simulink model "INP_test"  (R2024b)
settings: Solver=VariableStepAuto  StartTime=0.0  StopTime=10.0  RelTol=1e-3
libraries: simulink x1, INP x1
settings Model: Creator=blatak  LastModifiedBy=blatak

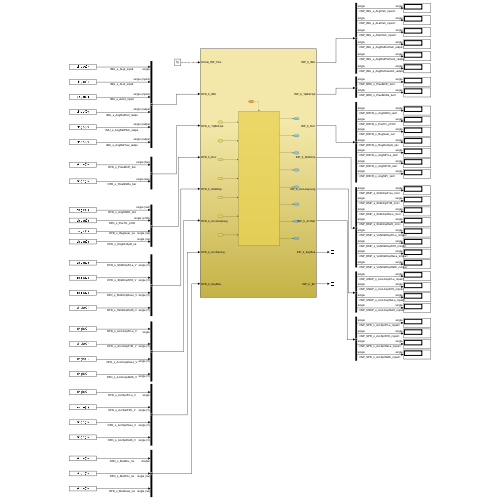
[thumbnail: Simulink's stored preview of the top-level diagram]
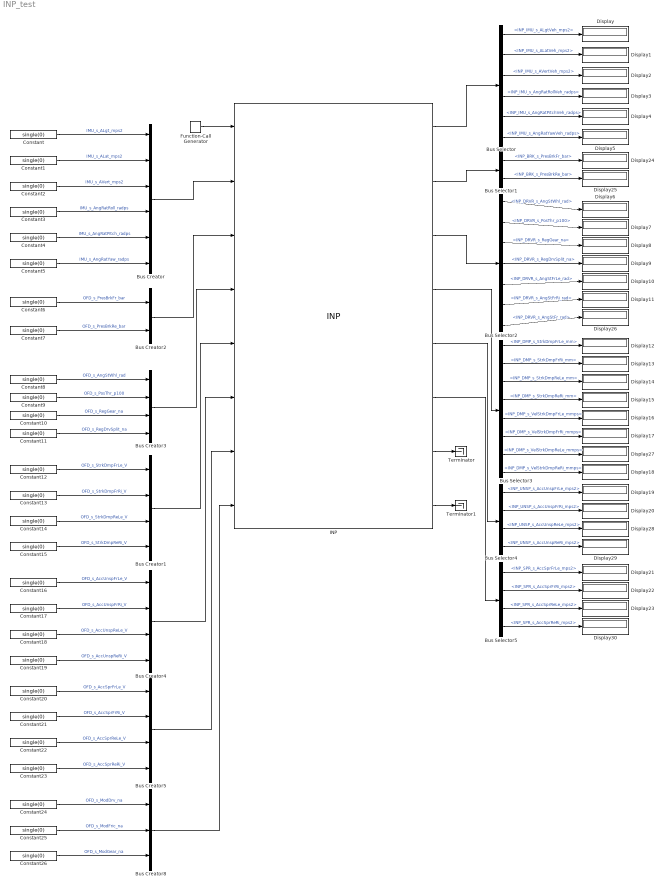
== system INP_test ==
  Bus Creator : BusCreator  Inputs=6  OutDataTypeStr=Bus: OFD_b_IMU
      settings: InheritFromInputs=off
  Bus Creator1 : BusCreator  Inputs=4  OutDataTypeStr=Bus: OFD_b_StrkDmp
      settings: InheritFromInputs=off
  Bus Creator2 : BusCreator  Inputs=2  OutDataTypeStr=Bus: OFD_b_TqBrkHyd
      settings: InheritFromInputs=off
  Bus Creator3 : BusCreator  Inputs=4  OutDataTypeStr=Bus: OFD_b_Drvr
      settings: InheritFromInputs=off
  Bus Creator4 : BusCreator  Inputs=4  OutDataTypeStr=Bus: OFD_b_AccUnsp
      settings: InheritFromInputs=off
  Bus Creator5 : BusCreator  Inputs=4  OutDataTypeStr=Bus: OFD_b_AccSpr
      settings: InheritFromInputs=off
  Bus Creator8 : BusCreator  Inputs=3  OutDataTypeStr=Bus: OFD_b_KeyBoa
      settings: InheritFromInputs=off
  Bus Selector : BusSelector  OutputSignals=INP_IMU_s_ALgtVeh_mps2,INP_IMU_s_ALatVeh_mps2,INP_IMU_s_AVertVeh_mps2,INP_IMU_s_AngRatRollVeh_radps,INP_IMU_s_AngRatPitchVeh_radps,INP_IMU_s_AngRatYawVeh_radps
  Bus Selector1 : BusSelector  OutputSignals=INP_BRK_s_PresBrkFr_bar,INP_BRK_s_PresBrkRe_bar
  Bus Selector2 : BusSelector  OutputSignals=INP_DRVR_s_AngStWhl_rad,INP_DRVR_s_PosThr_p100,INP_DRVR_s_RegGear_na,INP_DRVR_s_RegDrvSplit_na,INP_DRVR_s_AngStFrLe_rad,INP_DRVR_s_AngStFrRi_rad,INP_DRVR_s_AngStFr_rad
  Bus Selector3 : BusSelector  OutputSignals=INP_DMP_s_StrkDmpFrLe_mm,INP_DMP_s_StrkDmpFrRi_mm,INP_DMP_s_StrkDmpReLe_mm,INP_DMP_s_StrkDmpReRi_mm,INP_DMP_s_VelStrkDmpFrLe_mmps,INP_DMP_s_VelStrkDmpFrRi_mmps,INP_DMP_s_VelStrkDmpReLe_mmps,INP_DMP_s_VelStrkDmpReRi_mmps
  Bus Selector4 : BusSelector  OutputSignals=INP_UNSP_s_AccUnspFrLe_mps2,INP_UNSP_s_AccUnspFrRi_mps2,INP_UNSP_s_AccUnspReLe_mps2,INP_UNSP_s_AccUnspReRi_mps2
  Bus Selector5 : BusSelector  OutputSignals=INP_SPR_s_AccSprFrLe_mps2,INP_SPR_s_AccSprFrRi_mps2,INP_SPR_s_AccSprReLe_mps2,INP_SPR_s_AccSprReRi_mps2
  Constant{,1..26} (27 alike) : Constant  Value=single(0)
  Display{,1..30} (31 alike) : Display
  Function-Call Generator : simulink/Ports & Subsystems/Function-Call Generator  sample_time=0.005  numberOfIterations=1  DisallowWideOutput=off
  INP : INP/INP  SystemSampleTime=-1  VariantActivationTime=update diagram  AllowFlexibleInterface=on  Latency=0  AutoFrameSizeCalculation=off
  Terminator : Terminator
  Terminator1 : Terminator
  wires:
  Function-Call Generator/1 -> INP/1
  Constant19/1 -> Bus Creator4/4  "OFD_s_AccUnspReRi_V"
  Constant13/1 -> Bus Creator1/2  "OFD_s_StrkDmpFrRi_V"
  Constant14/1 -> Bus Creator1/3  "OFD_s_StrkDmpReLe_V"
  Constant3/1 -> Bus Creator/4  "IMU_s_AngRatRoll_radps"
  Constant1/1 -> Bus Creator/2  "IMU_s_ALat_mps2"
  Constant5/1 -> Bus Creator/6  "IMU_s_AngRatYaw_radps"
  Constant10/1 -> Bus Creator3/3  "OFD_s_RegGear_na"
  Bus Creator1/1 -> INP/5
  Bus Creator4/1 -> INP/6
  Constant/1 -> Bus Creator/1  "IMU_s_ALgt_mps2"
  Constant15/1 -> Bus Creator1/4  "OFD_s_StrkDmpReRi_V"
  Constant2/1 -> Bus Creator/3  "IMU_s_AVert_mps2"
  Constant25/1 -> Bus Creator8/2  "OFD_s_ModFric_na"
  Constant4/1 -> Bus Creator/5  "IMU_s_AngRatPitch_radps"
  Bus Creator3/1 -> INP/4
  Bus Creator2/1 -> INP/3
  Constant8/1 -> Bus Creator3/1  "OFD_s_AngStWhl_rad"
  Constant6/1 -> Bus Creator2/1  "OFD_s_PresBrkFr_bar"
  Constant11/1 -> Bus Creator3/4  "OFD_s_RegDrvSplit_na"
  Bus Creator/1 -> INP/2
  Constant12/1 -> Bus Creator1/1  "OFD_s_StrkDmpFrLe_V"
  Constant24/1 -> Bus Creator8/1  "OFD_s_ModDrv_na"
  Constant16/1 -> Bus Creator4/1  "OFD_s_AccUnspFrLe_V"
  Constant22/1 -> Bus Creator5/3  "OFD_s_AccSprReLe_V"
  Bus Creator5/1 -> INP/7
  Constant18/1 -> Bus Creator4/3  "OFD_s_AccUnspReLe_V"
  Constant21/1 -> Bus Creator5/2  "OFD_s_AccSprFrRi_V"
  Constant7/1 -> Bus Creator2/2  "OFD_s_PresBrkRe_bar"
  Constant20/1 -> Bus Creator5/1  "OFD_s_AccSprFrLe_V"
  Constant9/1 -> Bus Creator3/2  "OFD_s_PosThr_p100"
  Constant17/1 -> Bus Creator4/2  "OFD_s_AccUnspFrRi_V"
  Constant23/1 -> Bus Creator5/4  "OFD_s_AccSprReRi_V"
  Bus Creator8/1 -> INP/8
  INP/1 -> Bus Selector/1
  INP/2 -> Bus Selector1/1
  INP/3 -> Bus Selector2/1
  INP/4 -> Bus Selector3/1
  INP/5 -> Bus Selector4/1
  INP/6 -> Bus Selector5/1
  INP/7 -> Terminator/1
  INP/8 -> Terminator1/1
  Bus Selector1/1 -> Display24/1  "<INP_BRK_s_PresBrkFr_bar>"
  Bus Selector/1 -> Display/1  "<INP_IMU_s_ALgtVeh_mps2>"
  Bus Selector/2 -> Display1/1  "<INP_IMU_s_ALatVeh_mps2>"
  Bus Selector/3 -> Display2/1  "<INP_IMU_s_AVertVeh_mps2>"
  Bus Selector/4 -> Display3/1  "<INP_IMU_s_AngRatRollVeh_radps>"
  Bus Selector/5 -> Display4/1  "<INP_IMU_s_AngRatPitchVeh_radps>"
  Bus Selector/6 -> Display5/1  "<INP_IMU_s_AngRatYawVeh_radps>"
  Bus Selector1/2 -> Display25/1  "<INP_BRK_s_PresBrkRe_bar>"
  Bus Selector2/1 -> Display6/1  "<INP_DRVR_s_AngStWhl_rad>"
  Bus Selector2/2 -> Display7/1  "<INP_DRVR_s_PosThr_p100>"
  Bus Selector2/3 -> Display8/1  "<INP_DRVR_s_RegGear_na>"
  Bus Selector2/4 -> Display9/1  "<INP_DRVR_s_RegDrvSplit_na>"
  Bus Selector2/5 -> Display10/1  "<INP_DRVR_s_AngStFrLe_rad>"
  Bus Selector2/6 -> Display11/1  "<INP_DRVR_s_AngStFrRi_rad>"
  Bus Selector2/7 -> Display26/1  "<INP_DRVR_s_AngStFr_rad>"
  Bus Selector3/1 -> Display12/1  "<INP_DMP_s_StrkDmpFrLe_mm>"
  Bus Selector3/2 -> Display13/1  "<INP_DMP_s_StrkDmpFrRi_mm>"
  Bus Selector3/3 -> Display14/1  "<INP_DMP_s_StrkDmpReLe_mm>"
  Bus Selector3/4 -> Display15/1  "<INP_DMP_s_StrkDmpReRi_mm>"
  Bus Selector3/5 -> Display16/1  "<INP_DMP_s_VelStrkDmpFrLe_mmps>"
  Bus Selector3/6 -> Display17/1  "<INP_DMP_s_VelStrkDmpFrRi_mmps>"
  Bus Selector3/7 -> Display27/1  "<INP_DMP_s_VelStrkDmpReLe_mmps>"
  Bus Selector3/8 -> Display18/1  "<INP_DMP_s_VelStrkDmpReRi_mmps>"
  Bus Selector4/1 -> Display19/1  "<INP_UNSP_s_AccUnspFrLe_mps2>"
  Bus Selector4/2 -> Display20/1  "<INP_UNSP_s_AccUnspFrRi_mps2>"
  Bus Selector4/3 -> Display28/1  "<INP_UNSP_s_AccUnspReLe_mps2>"
  Bus Selector4/4 -> Display29/1  "<INP_UNSP_s_AccUnspReRi_mps2>"
  Bus Selector5/1 -> Display21/1  "<INP_SPR_s_AccSprFrLe_mps2>"
  Bus Selector5/2 -> Display22/1  "<INP_SPR_s_AccSprFrRi_mps2>"
  Bus Selector5/3 -> Display23/1  "<INP_SPR_s_AccSprReLe_mps2>"
  Bus Selector5/4 -> Display30/1  "<INP_SPR_s_AccSprReRi_mps2>"
  Constant26/1 -> Bus Creator8/3  "OFD_s_ModGear_na"
